simulink model "simulink_model_file"  (R2024b)
settings: Solver=ode45  StartTime=0.0  StopTime=60  MaxStep=0.005  RelTol=1e-3  EnableMultiTasking=on
values from neighbouring files (symbols this model uses):
  c = c2    (= 142.11)    [ProjectB_MATLAB.m]
  k = 3074    [ProjectB_MATLAB.m]
  m = 17.65+0.6    (= 18.25)    [ProjectB_MATLAB.m]
  m0 = 0.6    [ProjectB_MATLAB.m]
  v0 = -0.0037    [ProjectB_MATLAB.m]
  w = d(i)    [ProjectB_MATLAB.m]
  x0 = 0.0026    [ProjectB_MATLAB.m]
settings Model: Creator=hhaz001  LastModifiedBy=mjamz
settings SolverCC: AlgebraicLoopSolver=TrustRegion
settings DataIOCC: SaveFormat=Array  SaveOutput=off  ReturnWorkspaceOutputs=off
settings OptimizationCC: LifeSpan=inf
settings DebuggingCC: SolverPrmCheckMsg=warning  UnconnectedInputMsg=warning  UnconnectedOutputMsg=warning  UnconnectedLineMsg=warning  AllowSymbolicDim=off  SFUnexpectedBacktrackingDiag=warning  SFNoUnconditionalDefaultTransitionDiag=warning  SFExecutionAtInitializationDiag=none  ArithmeticOperatorsInVariantConditions=warning
settings HardwareCC: ProdBitPerPointer=32  ProdBitPerSizeT=32  ProdBitPerPtrDiffT=32  ProdLargestAtomicFloat=None  ProdIntDivRoundTo=Undefined  ProdEndianess=Unspecified  ProdWordSize=32  ProdHWDeviceType=32-bit Generic
settings ModelReferenceCC: EnableRefExpFcnMdlSchedulingChecks=on  PropagateSignalLabelsOutOfModel=off
settings SFSimCC: SimUseLocalCustomCode=off  CustomCodeUndefinedFunction=UseInterfaceOnly
settings RTWCC: RTWUseLocalCustomCode=off  GPUComputeCapability=3.5  DLArmComputeVersion=19.05
settings CodeAppCC: StateflowObjectComments=on
settings GRTTargetCC: TargetLangStandard=C89/C90 (ANSI)
settings ConfigComp: CovMetricSettings=dw  CovSaveCumulativeToWorkspaceVar=on  CovSaveSingleToWorkspaceVar=on  CovExternalEMLEnable=off  CovSFcnEnable=off

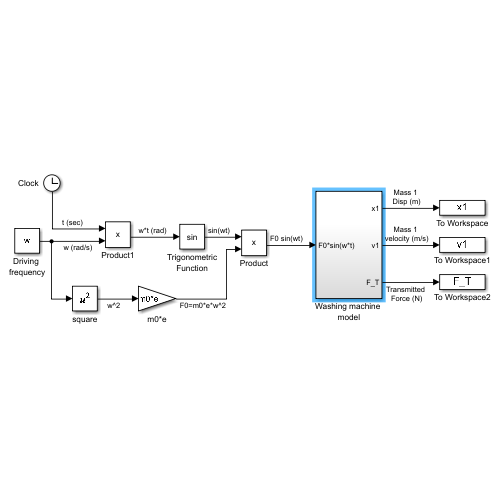
[thumbnail: Simulink's stored preview of the top-level diagram]
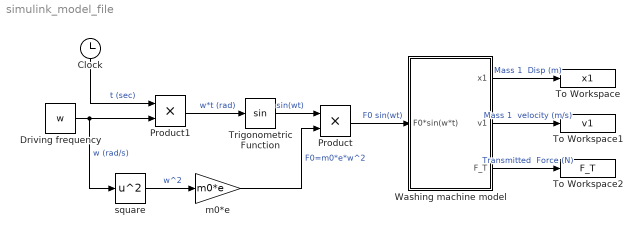
== system simulink_model_file ==
  Clock : Clock
  Driving frequency : Constant  Value=w
  Product : Product
  Product1 : Product
  To Workspace : ToWorkspace  VariableName=x1  SampleTime=-1
  To Workspace1 : ToWorkspace  VariableName=v1  SampleTime=-1
  To Workspace2 : ToWorkspace  VariableName=F_T  SampleTime=-1
  Trigonometric Function : Trigonometry
  Washing machine model : Subsystem
  m0*e : Gain  Gain=m0*e
  square : Math  Operator=square  SignedPower=on
  wires:
  Washing machine model/3(F_T) -> To Workspace2/1  "Transmitted  Force (N)"
  Washing machine model/1(x1) -> To Workspace/1  "Mass 1  Disp (m)"
  Product/1 -> Washing machine model/1(F0*sin(w*t))  "F0 sin(wt)"
  Driving frequency/1 -> square/1, Product1/2  "w (rad/s)"
  Trigonometric Function/1 -> Product/1  "sin(wt)"
  Product1/1 -> Trigonometric Function/1  "w*t (rad)"
  Clock/1 -> Product1/1  "t (sec)"
  square/1 -> m0*e/1  "w^2"
  m0*e/1 -> Product/2  "F0=m0*e*w^2"
  Washing machine model/2(v1) -> To Workspace1/1  "Mass 1  velocity (m/s)"

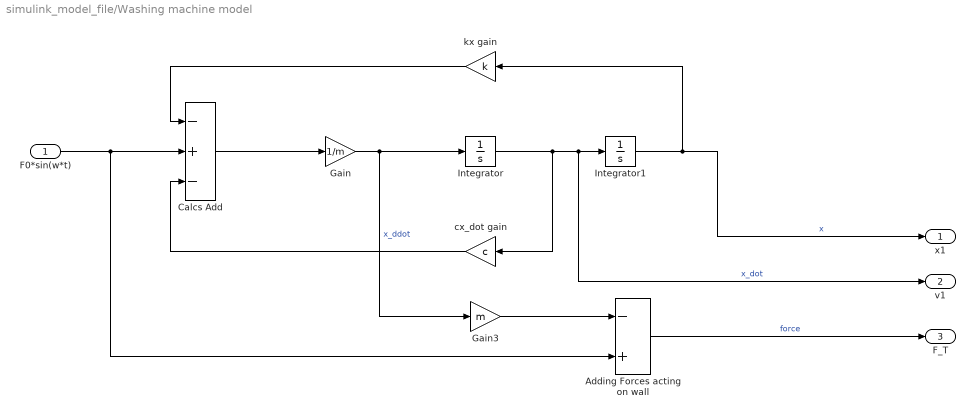
== system simulink_model_file/Washing machine model ==
  F0*sin(w*t) : Inport
  Adding Forces acting on wall : Sum  Inputs=-+
  Calcs Add : Sum  Inputs=-+-
  Gain : Gain  Gain=1/m
  Gain3 : Gain  Gain=m
  Integrator : Integrator  InitialCondition=v0
  Integrator1 : Integrator  InitialCondition=x0
  cx_dot gain : Gain  Gain=c
  kx gain : Gain  Gain=k
  x1 : Outport  VectorParamsAs1DForOutWhenUnconnected=off
  v1 : Outport  Port=2  VectorParamsAs1DForOutWhenUnconnected=off
  F_T : Outport  Port=3  VectorParamsAs1DForOutWhenUnconnected=off
  wires:
  Gain/1 -> Gain3/1, Integrator/1  "x_ddot"
  Integrator/1 -> cx_dot gain/1, v1/1, Integrator1/1  "x_dot"
  Integrator1/1 -> kx gain/1, x1/1  "x"
  Calcs Add/1 -> Gain/1
  kx gain/1 -> Calcs Add/1
  cx_dot gain/1 -> Calcs Add/3
  F0*sin(w*t)/1 -> Adding Forces acting on wall/2, Calcs Add/2
  Gain3/1 -> Adding Forces acting on wall/1
  Adding Forces acting on wall/1 -> F_T/1  "force"
